simulink model "IFF_Heterogenous_simu"  (R2019b)
settings: Solver=FixedStepAuto  StartTime=0.0  StopTime=100  FixedStep=0.001  RelTol=1e-3
values from neighbouring files (symbols this model uses):
  Af = F.A    [IFF_Heterogenous.m]
  Ag = SCM.A    [IFF_Heterogenous.m]
  B_k = inv(Nx)*R*L    [IFF_Heterogenous.m]
  Bf = F.B    [IFF_Heterogenous.m]
  Bg = [0 0 ... (first row only)    [IFF_Heterogenous.m]
  C_k = F*S*(inv(Mx))'    [IFF_Heterogenous.m]
  Cf = F.C    [IFF_Heterogenous.m]
  d = 0.2    [IFF_Heterogenous.m]
  D_k = zeros(size(C_k,1),size(B_k,2))    [IFF_Heterogenous.m]
  Df = F.D    [IFF_Heterogenous.m]
  Dr = diag(rmax)    [IFF_Heterogenous.m]
  Du = diag(umax)    [IFF_Heterogenous.m]
  st = 1    [IFF_Heterogenous.m]
  vt = -1:st:1    [IFF_Heterogenous.m]
undefined symbols (not defined in the file or in its folder): A_k
libraries: dspsigattribs x4
settings Model: Creator=AA  LastModifiedBy=AA

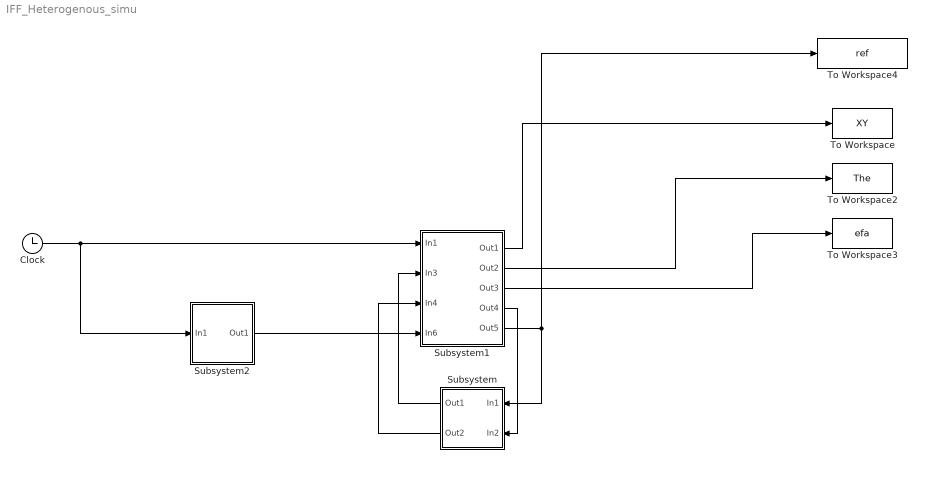
== system IFF_Heterogenous_simu ==
  Clock : Clock
  Subsystem : Subsystem
  Subsystem1 : Subsystem
  Subsystem2 : Subsystem
  To Workspace : ToWorkspace  VariableName=XY  SaveFormat=Timeseries  SampleTime=-1
  To Workspace2 : ToWorkspace  VariableName=The  SaveFormat=Timeseries  SampleTime=-1
  To Workspace3 : ToWorkspace  VariableName=efa  SaveFormat=Timeseries  SampleTime=0.001
  To Workspace4 : ToWorkspace  VariableName=ref  SaveFormat=Timeseries  SampleTime=-1
  wires:
  Clock/1 -> Subsystem2/1(In1), Subsystem1/1(In1)
  Subsystem/1(Out1) -> Subsystem1/2(In3)
  Subsystem/2(Out2) -> Subsystem1/3(In4)
  Subsystem1/2(Out2) -> To Workspace2/1
  Subsystem1/3(Out3) -> To Workspace3/1
  Subsystem1/4(Out4) -> Subsystem/2(In2)
  Subsystem1/5(Out5) -> To Workspace4/1, Subsystem/1(In1)
  Subsystem2/1(Out1) -> Subsystem1/4(In6)
  Subsystem1/1(Out1) -> To Workspace/1

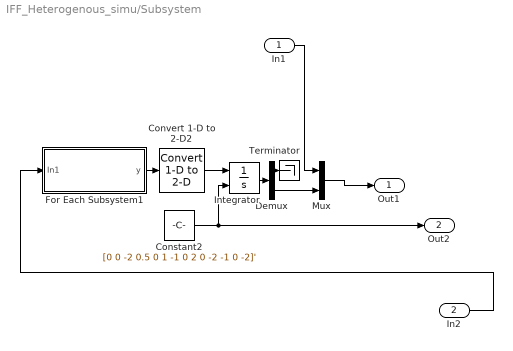
== system IFF_Heterogenous_simu/Subsystem ==
  In1 : Inport
  In2 : Inport  Port=2
  Constant2 : Constant  Value=[0 0 -2 0.5 0 1 -1 0 2 0 -2 -1 0 -2]'  SampleTime=0.001
  Convert 1-D to 2-D2 : dspsigattribs/Convert 1-D to 2-D  M=14  N=1  frameBasedOut=off
      settings: SourceProductName=DSP System Toolbox  SourceProductBaseCode=DS
  Demux : Demux  Outputs=[2 12]
  For Each Subsystem1 : Subsystem  TreatAsAtomicUnit=on
  Integrator : Integrator  InitialConditionSource=external
  Mux : Mux  Inputs=[2 12]
  Terminator : Terminator
  Out1 : Outport
  Out2 : Outport  Port=2
  wires:
  Constant2/1 -> Out2/1, Integrator/2
  In2/1 -> For Each Subsystem1/1(In1)
  Demux/1 -> Terminator/1
  For Each Subsystem1/1(y) -> Convert 1-D to 2-D2/1
  Convert 1-D to 2-D2/1 -> Integrator/1
  Integrator/1 -> Demux/1
  In1/1 -> Mux/1
  Mux/1 -> Out1/1
  Demux/2 -> Mux/2

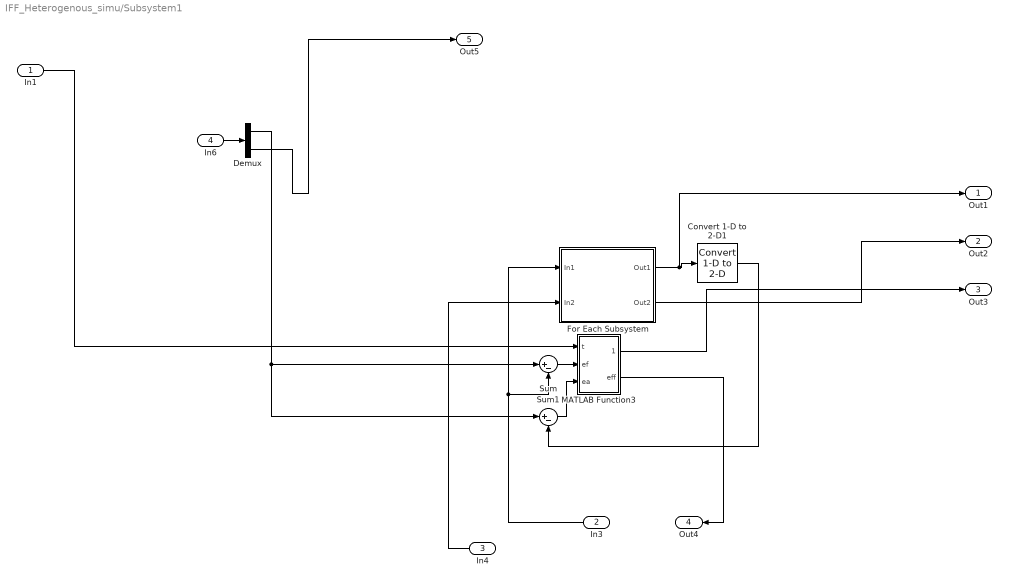
== system IFF_Heterogenous_simu/Subsystem1 ==
  In1 : Inport
  In3 : Inport  Port=2
  In4 : Inport  Port=3
  In6 : Inport  Port=4
  Convert 1-D to 2-D1 : dspsigattribs/Convert 1-D to 2-D  M=14  N=1  frameBasedOut=off
      settings: SourceProductName=DSP System Toolbox  SourceProductBaseCode=DS
  Demux : Demux  Outputs=[14 2]
  For Each Subsystem : Subsystem  TreatAsAtomicUnit=on
  MATLAB Function3 : MATLAB Function  TreatAsAtomicUnit=on
  Sum : Sum  Inputs=|+-
  Sum1 : Sum  Inputs=|+-
  Out1 : Outport
  Out2 : Outport  Port=2
  Out3 : Outport  Port=3
  Out4 : Outport  Port=4
  Out5 : Outport  Port=5
  wires:
  Demux/1 -> Sum1/1, Sum/1
  In1/1 -> MATLAB Function3/1(t)
  Convert 1-D to 2-D1/1 -> Sum1/2
  For Each Subsystem/1(Out1) -> Out1/1, Convert 1-D to 2-D1/1
  For Each Subsystem/2(Out2) -> Out2/1
  Sum1/1 -> MATLAB Function3/3(ea)
  In3/1 -> For Each Subsystem/1(In1), Sum/2
  MATLAB Function3/1(L2norm_efa) -> Out3/1
  Sum/1 -> MATLAB Function3/2(ef)
  MATLAB Function3/2(eff) -> Out4/1
  In4/1 -> For Each Subsystem/2(In2)
  In6/1 -> Demux/1
  Demux/2 -> Out5/1

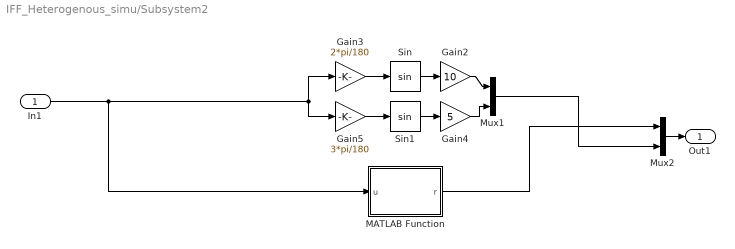
== system IFF_Heterogenous_simu/Subsystem2 ==
  In1 : Inport
  Gain2 : Gain  Gain=10
  Gain3 : Gain  Gain=2*pi/180
  Gain4 : Gain  Gain=5
  Gain5 : Gain  Gain=3*pi/180
  MATLAB Function : MATLAB Function  TreatAsAtomicUnit=on
  Mux1 : Mux  Inputs=2
  Mux2 : Mux  Inputs=[14 2]
  Sin : Trigonometry
  Sin1 : Trigonometry
  Out1 : Outport
  wires:
  Gain5/1 -> Sin1/1
  Sin1/1 -> Gain4/1
  Gain2/1 -> Mux1/1
  Sin/1 -> Gain2/1
  Gain4/1 -> Mux1/2
  Gain3/1 -> Sin/1
  Mux1/1 -> Mux2/2
  MATLAB Function/1(r) -> Mux2/1
  Mux2/1 -> Out1/1
  In1/1 -> MATLAB Function/1(u), Gain3/1, Gain5/1

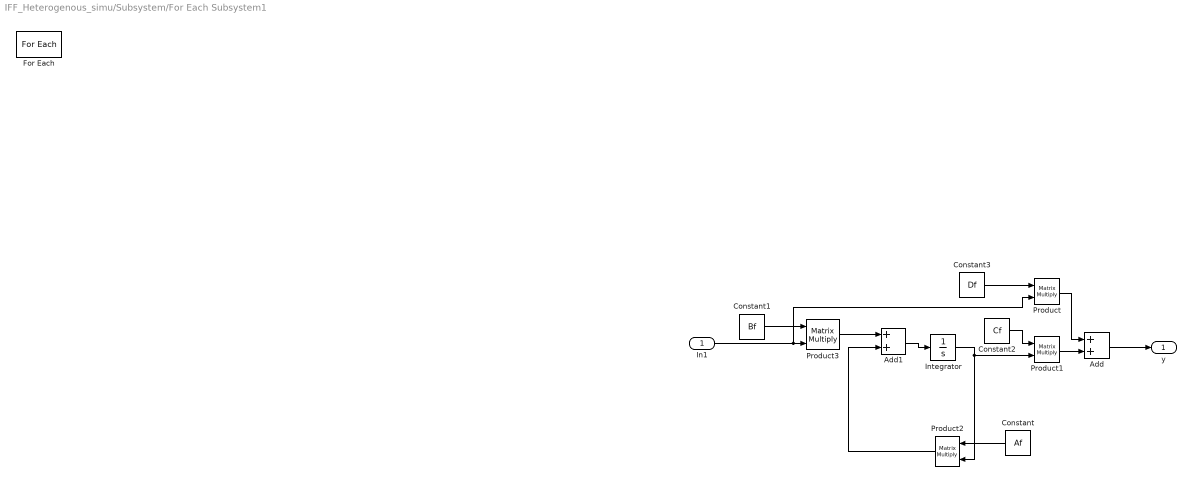
== system IFF_Heterogenous_simu/Subsystem/For Each Subsystem1 ==
  In1 : Inport  Partition=on  PartitionDimension=1  PartitionWidth=2  PartitionOffset=0
  Add : Sum
  Add1 : Sum
  Constant : Constant  Value=Af
  Constant1 : Constant  Value=Bf
  Constant2 : Constant  Value=Cf
  Constant3 : Constant  Value=Df
  For Each : ForEach  DisableCoverage=on
  Integrator : Integrator
  Product{,1..3} (4 alike) : Product  Multiplication=Matrix(*)
  y : Outport  ConcatenationDimension=2  VectorParamsAs1DForOutWhenUnconnected=off
  wires:
  Add/1 -> y/1
  In1/1 -> Product/2, Product3/2
  Product/1 -> Add/1
  Constant2/1 -> Product1/1
  Constant/1 -> Product2/1
  Integrator/1 -> Product1/2, Product2/2
  Constant1/1 -> Product3/1
  Add1/1 -> Integrator/1
  Product1/1 -> Add/2
  Product3/1 -> Add1/1
  Constant3/1 -> Product/1
  Product2/1 -> Add1/2

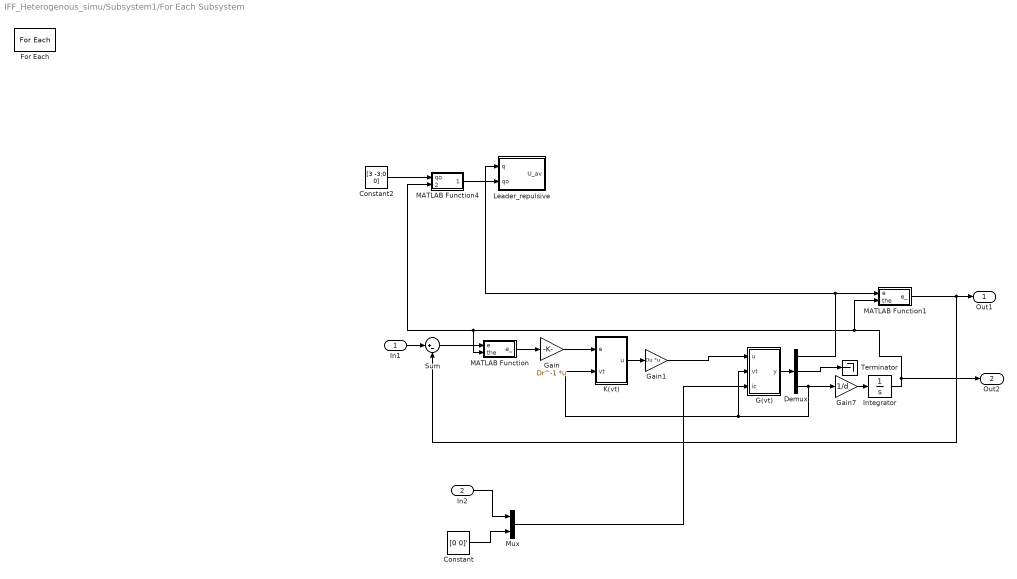
== system IFF_Heterogenous_simu/Subsystem1/For Each Subsystem ==
  In1 : Inport  Partition=on  PartitionDimension=1  PartitionWidth=2  PartitionOffset=0
  In2 : Inport  Port=2  Partition=on  PartitionDimension=1  PartitionWidth=2  PartitionOffset=0
  Constant : Constant  Value=[0 0]'
  Constant2 : Constant  Value=[3 -3;0 0]  SampleTime=0.01
  Demux : Demux  Outputs=[2 1 1]
  For Each : ForEach  DisableCoverage=on
  G(vt) : Subsystem
  Gain : Gain  Gain=Dr^-1  Multiplication=Matrix(K*u) (u vector)
  Gain1 : Gain  Gain=Du  Multiplication=Matrix(K*u) (u vector)
  Gain7 : Gain  Gain=1/d
  Integrator : Integrator
  K(vt) : Subsystem
  Leader_repulsive : MATLAB Function  TreatAsAtomicUnit=on
  MATLAB Function : MATLAB Function  TreatAsAtomicUnit=on
  MATLAB Function1 : MATLAB Function  TreatAsAtomicUnit=on
  MATLAB Function4 : MATLAB Function  TreatAsAtomicUnit=on
  Mux : Mux  Inputs=2
  Sum : Sum  Inputs=|+-
  Terminator : Terminator
  Out1 : Outport  ConcatenationDimension=2  VectorParamsAs1DForOutWhenUnconnected=off
  Out2 : Outport  Port=2  ConcatenationDimension=2  VectorParamsAs1DForOutWhenUnconnected=off
  wires:
  Gain7/1 -> Integrator/1
  G(vt)/1(y) -> Demux/1
  MATLAB Function/1(e_) -> Gain/1
  MATLAB Function1/1(e_) -> Out1/1, Sum/2
  Demux/3 -> Gain7/1, K(vt)/2(vt), G(vt)/2(vt)
  Demux/2 -> Terminator/1
  In1/1 -> Sum/1
  In2/1 -> Mux/1
  Constant/1 -> Mux/2
  Mux/1 -> G(vt)/3(ic)
  Gain1/1 -> G(vt)/1(u)
  Sum/1 -> MATLAB Function/1(e)
  K(vt)/1(u) -> Gain1/1
  Gain/1 -> K(vt)/1(e)
  Demux/1 -> Leader_repulsive/1(q), MATLAB Function1/1(e)
  Constant2/1 -> MATLAB Function4/1(qo)
  MATLAB Function4/1(qo_) -> Leader_repulsive/2(qo)
  Integrator/1 -> Out2/1, MATLAB Function1/2(the), MATLAB Function4/2(the), MATLAB Function/2(the)

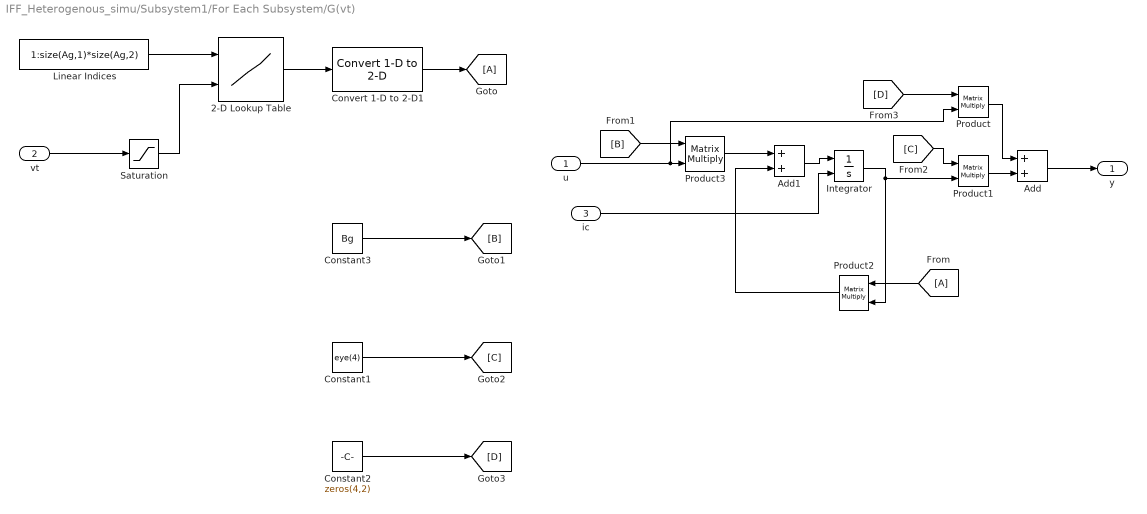
== system IFF_Heterogenous_simu/Subsystem1/For Each Subsystem/G(vt) ==
  u : Inport
  vt : Inport  Port=2
  ic : Inport  Port=3
  2-D Lookup Table : Lookup_n-D  BreakpointsForDimension1=1:size(Ag,1)*size(Ag,2)  BreakpointsForDimension2=[-1:st:1]  Table=reshape(Ag,[size(Ag,1)*size(Ag,2), length(vt)'])  InternalRulePriority=Speed  RndMeth=Simplest  InputSameDT=on
  Add : Sum
  Add1 : Sum
  Constant1 : Constant  Value=eye(4)
  Constant2 : Constant  Value=zeros(4,2)
  Constant3 : Constant  Value=Bg
  Convert 1-D to 2-D1 : dspsigattribs/Convert 1-D to 2-D  M=size(Ag,1)  N=size(Ag,2)  frameBasedOut=off
      settings: SourceProductName=DSP System Toolbox  SourceProductBaseCode=DS
  Integrator : Integrator  InitialConditionSource=external
  Linear Indices : Constant  Value=1:size(Ag,1)*size(Ag,2)
  Product{,1..3} (4 alike) : Product  Multiplication=Matrix(*)
  Saturation : Saturate  UpperLimit=1  LowerLimit=-1
  y : Outport  VectorParamsAs1DForOutWhenUnconnected=off
  wires:
  Product3/1 -> Add1/1
  [B] -> Product3/1
  Add1/1 -> Integrator/1
  Product2/1 -> Add1/2
  Saturation/1 -> 2-D Lookup Table/2
  Linear Indices/1 -> 2-D Lookup Table/1
  2-D Lookup Table/1 -> Convert 1-D to 2-D1/1
  [C] -> Product1/1
  Integrator/1 -> Product1/2, Product2/2
  [D] -> Product/1
  Convert 1-D to 2-D1/1 -> [A]
  [A] -> Product2/1
  Product1/1 -> Add/2
  Product/1 -> Add/1
  u/1 -> Product/2, Product3/2
  Add/1 -> y/1
  Constant2/1 -> [D]
  Constant1/1 -> [C]
  vt/1 -> Saturation/1
  Constant3/1 -> [B]
  ic/1 -> Integrator/2

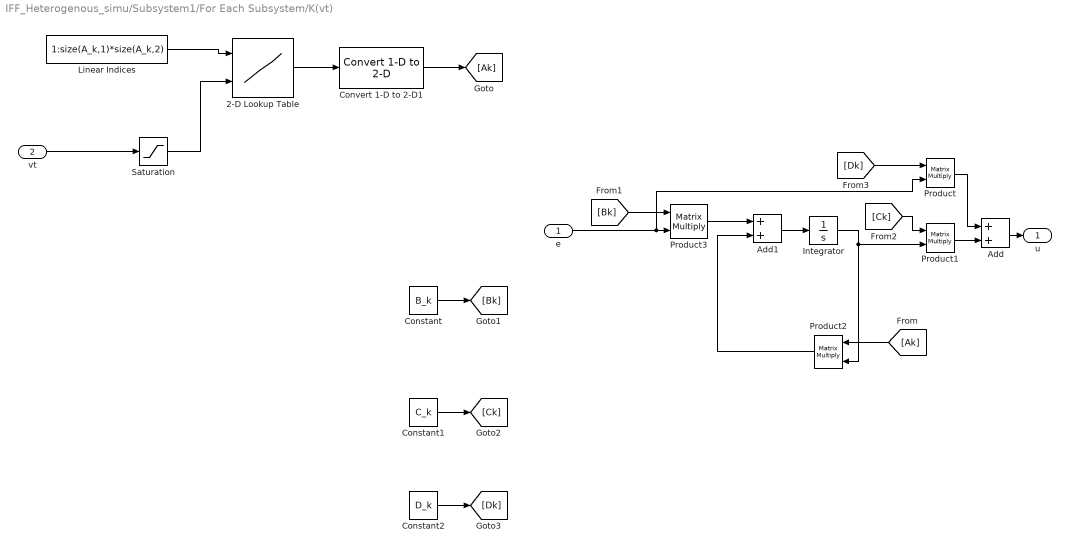
== system IFF_Heterogenous_simu/Subsystem1/For Each Subsystem/K(vt) ==
  e : Inport
  vt : Inport  Port=2
  2-D Lookup Table : Lookup_n-D  BreakpointsForDimension1=1:size(A_k,1)*size(A_k,2)  BreakpointsForDimension2=[-1:st:1]  BreakpointsForDimension3=[-1 1]  Table=reshape(A_k,[size(A_k,1)*size(A_k,2),length(vt)'])  InternalRulePriority=Speed  RndMeth=Simplest  InputSameDT=on
  Add : Sum
  Add1 : Sum
  Constant : Constant  Value=B_k
  Constant1 : Constant  Value=C_k
  Constant2 : Constant  Value=D_k
  Convert 1-D to 2-D1 : dspsigattribs/Convert 1-D to 2-D  M=size(A_k,1)  N=size(A_k,2)  frameBasedOut=off
      settings: SourceProductName=DSP System Toolbox  SourceProductBaseCode=DS
  Integrator : Integrator
  Linear Indices : Constant  Value=1:size(A_k,1)*size(A_k,2)
  Product{,1..3} (4 alike) : Product  Multiplication=Matrix(*)
  Saturation : Saturate  UpperLimit=1  LowerLimit=-1
  u : Outport  VectorParamsAs1DForOutWhenUnconnected=off
  wires:
  e/1 -> Product3/2, Product/2
  Product/1 -> Add/1
  Product1/1 -> Add/2
  [Ak] -> Product2/1
  Convert 1-D to 2-D1/1 -> [Ak]
  [Dk] -> Product/1
  Integrator/1 -> Product2/2, Product1/2
  [Ck] -> Product1/1
  vt/1 -> Saturation/1
  2-D Lookup Table/1 -> Convert 1-D to 2-D1/1
  Linear Indices/1 -> 2-D Lookup Table/1
  Product2/1 -> Add1/2
  Add1/1 -> Integrator/1
  [Bk] -> Product3/1
  Product3/1 -> Add1/1
  Saturation/1 -> 2-D Lookup Table/2
  Constant/1 -> [Bk]
  Constant1/1 -> [Ck]
  Constant2/1 -> [Dk]
  Add/1 -> u/1

== matlab function IFF_Heterogenous_simu/Subsystem2/MATLAB Function ==
  data: u input; r output
function r = fcn(u)
    t=u;
    y=zeros(14,1);
while 1    
    if t<=80
        break
    elseif t>80
        t= t-80;
    end
end

if t<=10
   y=[0 0 -0.5 1 0.5 1 -1.5 0 1.5 0 -0.5 -1 0.5 -1]';
elseif t>10 && t<=20
    y=[0 0 -1 1 1 1 -1 0 1 0 -1 -1 1 -1]';     
elseif t>20 && t<=30
    y=[0 0 -0.5 0 0.5 0 -1 0 1 0 -1.5 0 1.5 0]';   
elseif t>30 && t<=40
    y=[0 0 -0.5 0 0.5 0 0 1 0 -1 -1 0 1 0]';   
elseif t>40 && t<=50
       y=[0 0 -1 1 1 1 0 1 0 -1 -1 -1 1 -1]';       
elseif t>50 && t<=60
    y=[0 0 -0.5 0 0.5 0 0 1 0 -1 -1 0 1 0]';
elseif t>60 && t<=70
    y=[0 0 -0.5 0 0.5 0 -1 0 1 0 -1.5 0 1.5 0]';
elseif t>70 && t<=80
 y=[0 0 -0.5 0 0.5 0 0 1 0 -1 -1 0 1 0]';
end

r = y;

== matlab function IFF_Heterogenous_simu/Subsystem1/For Each Subsystem/MATLAB Function ==
  data: e input; e_ output; the input
function e_ = fcn(e,the)

e_ = [cos(the) sin(the);-sin(the) cos(the)]*e;

== matlab function IFF_Heterogenous_simu/Subsystem1/For Each Subsystem/MATLAB Function1 ==
  data: e input; e_ output; the input
function e_ = fcn(e,the)

e_ = [cos(the) -sin(the);sin(the) cos(the)]*e;

== matlab function IFF_Heterogenous_simu/Subsystem1/MATLAB Function3 ==
  settings: updateMethod=DISCRETE
  data: t input; ef input; L2norm_efa output; eff output; ea input
function [L2norm_efa,eff] = fcn(t,ef,ea)
L2norm_efa=0;
L2norm_eff=0;
eff=zeros(14,1);
L=zeros(14,14);
D=zeros(7,7);
D0=zeros(7,7);
p=rand(7,7);
 for i=1:7
    for j=1:7
       if  i~=j && p(i,j)>0.0
           D0(i,j)=1;
       end
    end
 end
 
D0(1,:)=zeros(1,7);
D0(2,5)=0;
D0(2,6)=0;
D0(2,7)=0;
D0(3,4)=0;
D0(3,6)=0;
D0(3,7)=0;
D0(4,3)=0;
D0(4,5)=0;
D0(4,7)=0;
D0(5,2)=0;
D0(5,4)=0;
D0(5,6)=0;
D0(6,2)=0;
D0(6,3)=0;
D0(6,5)=0;
D0(7,2)=0;
D0(7,3)=0;
D0(7,4)=0; 
 
slack=sum(D0,2);
for i=1:length(slack)
    if slack(i)==0
        slack(i)=1;
    end
end
D=diag(1./slack)*D0;
l=blkdiag(0,eye(6))-D;
L=kron(l,eye(2));
L2norm_efa=norm(L*ea,2);
eff=L*ef;
L2norm_eff=norm(L*ef,2);

== matlab function IFF_Heterogenous_simu/Subsystem1/For Each Subsystem/Leader_repulsive ==
  data: q input; qo input; U_av output
% Collision Avoidance Function
function U_av = fcn(q,qo)
uav=zeros(2,length(qo(1,:)));
for i=1:length(qo(1,:))
    if norm(q-qo(:,i))<2        
        uav(:,i)=[3.5*exp(-0.1*((q(1)-qo(1,i)/1)^2+(q(2)-qo(2,i)/1)^2))*(q(1)-qo(1,i)/1)
                  3.5*exp(-0.1*((q(1)-qo(1,i)/1)^2+(q(2)-qo(2,i)/1)^2))*(q(2)-qo(2,i)/1)];
    else
        uav(:,i)=[0;0];
    end
end
U_av=sum(uav,2);
end

== matlab function IFF_Heterogenous_simu/Subsystem1/For Each Subsystem/MATLAB Function4 ==
  data: qo input; qo_ output; the input
function qo_ = fcn(qo,the)
qo_=zeros(2,length(qo(1,:)));
for i=1:length(qo(1,:))
    qo_(:,i) = [cos(the) sin(the);-sin(the) cos(the)]*qo(:,i);
end
